simulink model "PID_PFL_3D_winds"  (R2022b)
settings: Solver=ode15s  StartTime=0.0  StopTime=0.8803  RelTol=1e-3
values from neighbouring files (symbols this model uses):
  theta1x_in = pinput(4 : 3 + n)    [Animation_3D.m]    (also in Constraint_3D_WCW.m = pinput(4 : 3+n); Cost_3D_WCW.m = pinput(4 : 3+n))
  theta1y_in = pinput(4 + n : 3 + 2*n)    [Animation_3D.m]    (also in Constraint_3D_WCW.m = pinput(4+n : 3+2*n); Cost_3D_WCW.m = pinput(4+n : 3+2*n))
  theta2_in = pinput(4 + 2*n : 3 + 3*n)    [Animation_3D.m]    (also in Constraint_3D_WCW.m = pinput(4+2*n : 3+3*n); Cost_3D_WCW.m = pinput(4+2*n : 3+3*n))
  timeVec = linspace(0, simTime, n)'    [Animation_3D.m]    (also in Main_3D_WCW.m = linspace(0, xmin(1), n)')
undefined symbols (not defined in the file or in its folder): sigbuilder_block, windSpeed
libraries: nesl_utility x6, sm_lib x4, slpidlib x3, simulink_extras x1
(part 2 of 2)

== matlab function PID_PFL_3D_winds/Subsystem/Determining Angular Accelerations  ==
  settings: updateMethod=DISCRETE
  data: theta1x input; ddtheta1x output; theta1y input; theta1z input; theta2 input; dtheta1x input; dtheta1y input; dtheta2 input; wind_torque1 input; wind_torque2 input; ddtheta1y output; ddtheta1z output; ddtheta2 output; F1 output; F2 output; F_brake output; torque_elbow input; torque_wrist_y input; dtheta1z input
function [ddtheta1x, ddtheta1y, ddtheta1z, ddtheta2, F1, F2, F_brake] = ...
    fcn(theta1x, theta1y, theta1z, theta2, dtheta1x, dtheta1y, dtheta2, ...
        wind_torque1, wind_torque2, torque_elbow, torque_wrist_y, dtheta1z)

% Robustified plant dynamics (safer numerics and torque saturation).
% Inputs/outputs kept identical to your original function.

%% ------------- User-tunable safety / debug params -------------------
debug = false;            % set true to print a few diagnostics (costly)
max_torque_elbow = 20;   % saturate elbow torque (Nm)
max_torque_wrist = 10;   % saturate wrist_y torque (Nm)
max_ddtheta = 1e4;       % hard clamp on accelerations (rad/s^2)
epsv = 1e-6;             % small numeric regularizer to denominators
% Increase viscous damping slightly to help stability:
b1 = 1.0;    % shoulder viscous damping (was 0.3)
b2 = 1.0;    % elbow viscous damping (was 0.3)

%% ------------- parameters (unchanged physics) ----------------------
m1 = 4.8; m2 = 4.8;
l1 = 1.0; l2 = 1.0;
lc1 = 0.5*l1; lc2 = 0.5*l2;
g = 9.81;

% inertias (thin rod approx)
I1 = (1/3)*m1*l1^2;
I2 = (1/3)*m2*l2^2;

%% ------------- clamp / sanitize inputs -----------------------------
% Protect against NaN incoming values:
if any(isnan([theta1x,theta1y,theta1z,theta2,dtheta1x,dtheta1y,dtheta2]))
    error('fcn: NaN in inputs');
end

% Saturate torques from controller (prevents impulses)
torque_elbow = min(max(torque_elbow, -max_torque_elbow), max_torque_elbow);
torque_wrist_y = min(max(torque_wrist_y, -max_torque_wrist), max_torque_wrist);

%% ------------- friction outputs for logging ------------------------
F1 = abs(b1 * dtheta1x);
F2 = abs(b2 * dtheta2);
F_brake = 0;

%% ------------- dynamics (structured but approximate) --------------
% 1) Elbow equation (more robust numerics)
D2 = I2 + m2*lc2^2 + epsv;

% gravity/coriolis approximations
g_term_elbow = m2*lc2*( g * sin(theta1x + theta2) );
% keep optional y-coupling zero (as before)
% C_elbow uses both shoulder velocities (approx)
C_elbow = m2 * l1 * lc2 * ( dtheta1x^2 + dtheta1y^2 ) * sin(theta2);

ddtheta2 = ( torque_elbow - b2*dtheta2 - C_elbow - g_term_elbow - wind_torque2 ) / D2;

% clamp ddtheta2 if it explodes
if ~isfinite(ddtheta2), ddtheta2 = sign(ddtheta2)*max_ddtheta; end
ddtheta2 = max(min(ddtheta2, max_ddtheta), -max_ddtheta);

% 2) Shoulder x (sagittal)
Dx = I1 + m1*lc1^2 + m2*( l1^2 + lc2^2 + 2*l1*lc2*cos(theta2) ) + epsv;
% coupling terms
couple_x = - m2*l1*lc2*( ddtheta2*cos(theta2) - dtheta2^2 * sin(theta2) );
grav_x = (m1*lc1 + m2*l1) * g * sin(theta1x) + m2*lc2*g * sin(theta1x + theta2);
fric_x = - b1 * dtheta1x;
tau_wind_x = wind_torque1;  % if wind acts about x
tau_sh_x = 0;               % no shoulder-x actuator here

ddtheta1x = ( tau_sh_x + tau_wind_x + fric_x + couple_x - grav_x ) / Dx;
if ~isfinite(ddtheta1x), ddtheta1x = 0; end
ddtheta1x = max(min(ddtheta1x, max_ddtheta), -max_ddtheta);

% 3) Shoulder y (out-of-plane) with actuator torque_wrist_y
Dy = I1 + m1*lc1^2 + m2*( l1^2 + lc2^2 + 2*l1*lc2*cos(theta2) ) + epsv;
couple_y = - m2*l1*lc2*( ddtheta2*cos(theta2) - dtheta2^2 * sin(theta2) );
grav_y = (m1*lc1 + m2*l1) * g * sin(theta1y) + m2*lc2*g * sin(theta1y + theta2);
fric_y = - b1 * dtheta1y;
tau_sh_y = torque_wrist_y;

ddtheta1y = ( tau_sh_y + wind_torque1 + fric_y + couple_y - grav_y ) / Dy;
if ~isfinite(ddtheta1y), ddtheta1y = 0; end
ddtheta1y = max(min(ddtheta1y, max_ddtheta), -max_ddtheta);

% 4) z rotation not modeled
ddtheta1z = 0;

%% final NaN/Inf guard
if any(~isfinite([ddtheta1x, ddtheta1y, ddtheta1z, ddtheta2]))
    % graceful fallback to zero accelerations if something still went wrong
    ddtheta1x = 0; ddtheta1y = 0; ddtheta1z = 0; ddtheta2 = 0;
%     warning('fcn: numerical trouble - returning zeros for accelerations');
end

%% debug prints (toggle by setting debug=true)
if debug
    fprintf('[fcn] t_e=%.3f t_wy=%.3f ddth2=%.3f ddth1x=%.3f ddth1y=%.3f\n', ...
        torque_elbow, torque_wrist_y, ddtheta2, ddtheta1x, ddtheta1y);
end

end
